simulink model "sfcndemo_ada_times_two"  (Simulink 6.0)
settings: Solver=FixedStepDiscrete  StartTime=0.0  StopTime=10.0  FixedStep=0.1  RelTol=1e-3
settings Model: Creator=The MathWorks Inc.  LastModifiedBy=batserve  ExtModeTrigMode=oneshot  ExtModeArmWhenConnect=off  ExtModeAutoUpdateStatusClock=off
settings DataIOCC: LimitDataPoints=off  StateSaveName=x  TimeSaveName=t  OutputSaveName=y
settings OptimizationCC: BlockReduction=off  BooleanDataType=off  InlineInvariantSignals=off
settings DebuggingCC: ConsistencyChecking=error  ArrayBoundsChecking=error  CheckExecutionContextPreStartOutputMsg=on  CheckExecutionContextRuntimeOutputMsg=on  SolverPrmCheckMsg=none
settings HardwareCC: TargetUnknown=on
settings RTWCC: SystemTargetFile=rt_ada_sim.tlc  MakeCommand=make_rtw -ada=gnat3.12a2 -v  TemplateMakefile=gnat_sim.tmf  RetainRTWFile=on  ProcessScript=rt_ada_sim_make_rtw_hook
settings STFCustomTargetCC: TargetFcnLib=ansi_tfl_tmw.mat  GenFloatMathFcnCalls=ANSI_C  ModelReferenceCompliant=off  CombineOutputUpdateFcns=on  MatFileLogging=on  SystemTargetFile=rt_ada_sim.tlc

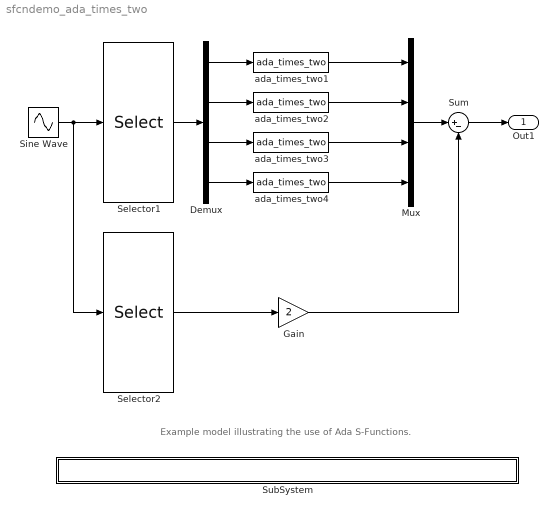
== system sfcndemo_ada_times_two ==
  note: Example model illustrating the use of Ada S-Functions.
  Demux : Demux  Outputs=[5, 4, 5, 1]
  Gain : Gain  Gain=2  SaturateOnIntegerOverflow=on
  Mux : Mux
  Selector1 : Selector  Elements=[3 4 5 6 7 14 15 1 2 10 11 12 13 8 9]  InputPortWidth=15
  Selector2 : Selector  Elements=[3 4 5 6 7 14 15 1 2 10 11 12 13 8 9]  InputPortWidth=15
  Sine Wave : Sin  Amplitude=[1:0.5:8]  Frequency=2*pi/10*[4.5:-0.25:1]  SampleTime=0.1
  SubSystem : Subsystem  PropExecContextAcrossSSBoundary=on
      settings: OpenFcn=evalin('base','edit(fullfile(matlabroot,''simulink'',''ada'',''examples'',''times_two'',''times_two.adb''))')
      mask Display: disp('matlabroot\simulink\ada\examples\times_two\times_two.adb');
  Sum : Sum  Inputs=|+-  SaturateOnIntegerOverflow=on  InputSameDT=on
  ada_times_two{1..4} (4 alike) : S-Function  FunctionName=ada_times_two
  Out1 : Outport
  wires:
  Sine Wave/1 -> Selector1/1, Selector2/1
  Selector1/1 -> Demux/1
  Demux/1 -> ada_times_two1/1
  Demux/2 -> ada_times_two2/1
  Demux/3 -> ada_times_two3/1
  Demux/4 -> ada_times_two4/1
  Selector2/1 -> Gain/1
  ada_times_two1/1 -> Mux/1
  ada_times_two2/1 -> Mux/2
  ada_times_two3/1 -> Mux/3
  ada_times_two4/1 -> Mux/4
  Sum/1 -> Out1/1
  Mux/1 -> Sum/1
  Gain/1 -> Sum/2

== system sfcndemo_ada_times_two/SubSystem ==
